simulink model "Main_Model_CB_EN_UEEE23112"  (R2025b)
settings: Solver=ode23t  StartTime=0.0  StopTime=25  MaxStep=1e-5  RelTol=1e-3  AbsTol=1e-4
values from neighbouring files (symbols this model uses):
  Tsc = 5e-5    (= 5e-05)    [Model_Parameters_CB_EN_U4EEE23112.m]
undefined symbols (not defined in the file or in its folder): dspblkCoreblockFVToolHelper, gcbh
libraries: nesl_utility x31, fl_lib x20, ee_lib x12, sdl_lib x4, batteryecm_lib x1, eePmsmFieldOrientedControl x1
(part 1 of 3)
settings Model: SimulationMode=accelerator  Creator=Hp  LastModifiedBy=Harish
settings SolverCC: AutoScaleAbsTol=off
settings ConfigComp: CovScope=ReferencedModels  CovMetricSettings=dzwe  CovHTMLOptions=-sRT=1 -sVT=0 -aTS=1 -agT=1 -bRG=1 -bTC=1 -hTR=0 -nFC=0 -nFD=0 -scm=1 -bcm=1 -xEv=0 -xEM=0 -req=1  CovEnableCumulative=off  CovCumulativeReport=on

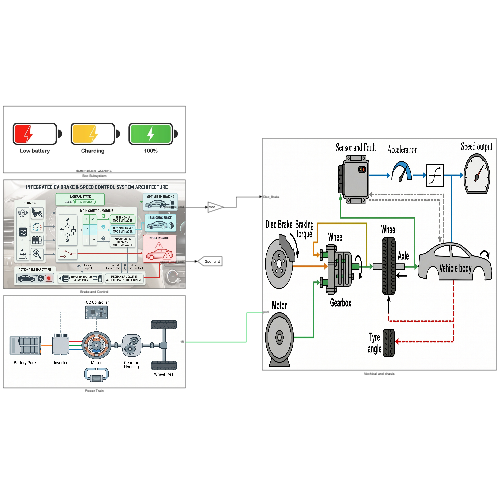
[thumbnail: Simulink's stored preview of the top-level diagram]
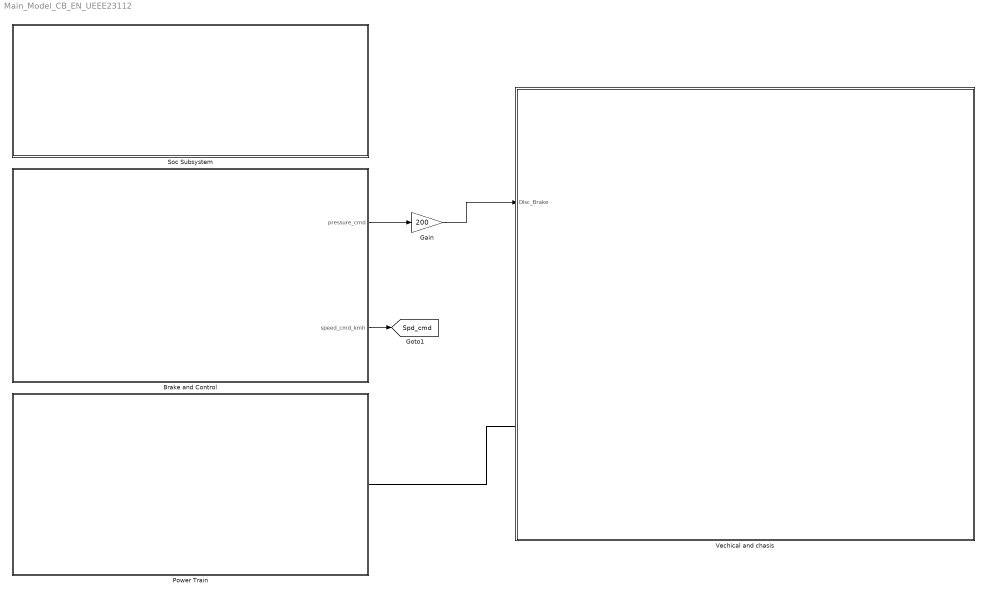
== system Main_Model_CB_EN_UEEE23112 ==
  Brake and Control : Subsystem
      mask Display: image('Brake_sub.png');
  Gain : Gain  Gain=200
  Power Train : Subsystem
      mask Display: image('Power_Train.png');
  Soc Subsystem : Subsystem
      mask Display: image('Soc.jpg');
  Vechical and chasis : Subsystem
      mask Display: image('Chasis.png');
  tag scope: Spd_cmd=global
  wires:
  Brake and Control/1(pressure_cmd) -> Gain/1
  Brake and Control/2(speed_cmd_kmh) -> [Spd_cmd]
  Gain/1 -> Vechical and chasis/1(Disc_Brake)
  connections:
  Power Train/RConn1 -- Vechical and chasis/LConn1

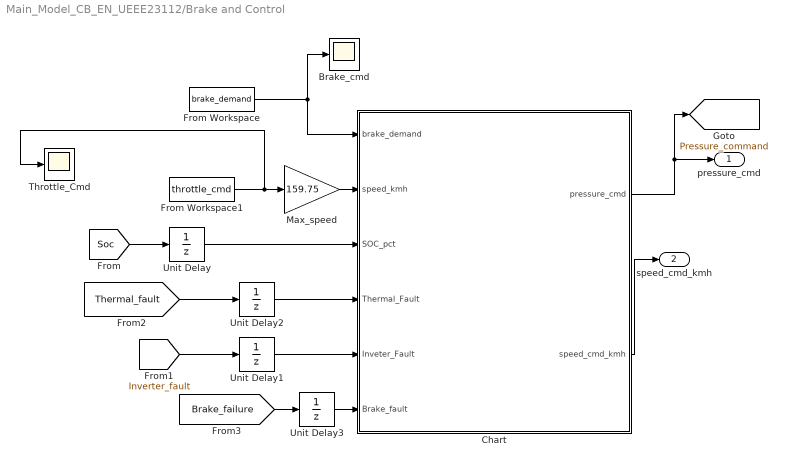
== system Main_Model_CB_EN_UEEE23112/Brake and Control ==
  Brake_cmd : Scope
      settings: ActiveDisplayYMinimum=-0.10624999999999997  ActiveDisplayYMaximum=0.95624999999999993  DataLoggingVariableName=ScopeData7
  Chart : Stateflow chart  TreatAsAtomicUnit=on
  From Workspace : FromWorkspace  VariableName=brake_demand  SampleTime=1e-4
  From Workspace1 : FromWorkspace  VariableName=throttle_cmd  SampleTime=1e-4
  Max_speed : Gain  Gain=159.75
  Throttle_Cmd : Scope
      settings: ActiveDisplayYMinimum=-0.049737499999999983  ActiveDisplayYMaximum=0.44763749999999997  DataLoggingVariableName=ScopeData8
  Unit Delay{,1..3} (4 alike) : UnitDelay  SampleTime=-1  HasFrameUpgradeWarning=on
  pressure_cmd : Outport
  speed_cmd_kmh : Outport  Port=2
  tag scope: Pressure_command=global
  wires:
  Chart/1(pressure_cmd) -> [Pressure_command], pressure_cmd/1
  Chart/2(speed_cmd_kmh) -> speed_cmd_kmh/1
  From Workspace1/1 -> Throttle_Cmd/1, Max_speed/1
  [Soc] -> Unit Delay/1
  From Workspace/1 -> Brake_cmd/1, Chart/1(brake_demand)
  Unit Delay/1 -> Chart/3(SOC_pct)
  Max_speed/1 -> Chart/2(speed_kmh)
  [Inverter_fault] -> Unit Delay1/1
  Unit Delay1/1 -> Chart/5(Inveter_Fault)
  [Thermal_fault] -> Unit Delay2/1
  Unit Delay2/1 -> Chart/4(Thermal_Fault)
  [Brake_failure] -> Unit Delay3/1
  Unit Delay3/1 -> Chart/6(Brake_fault)

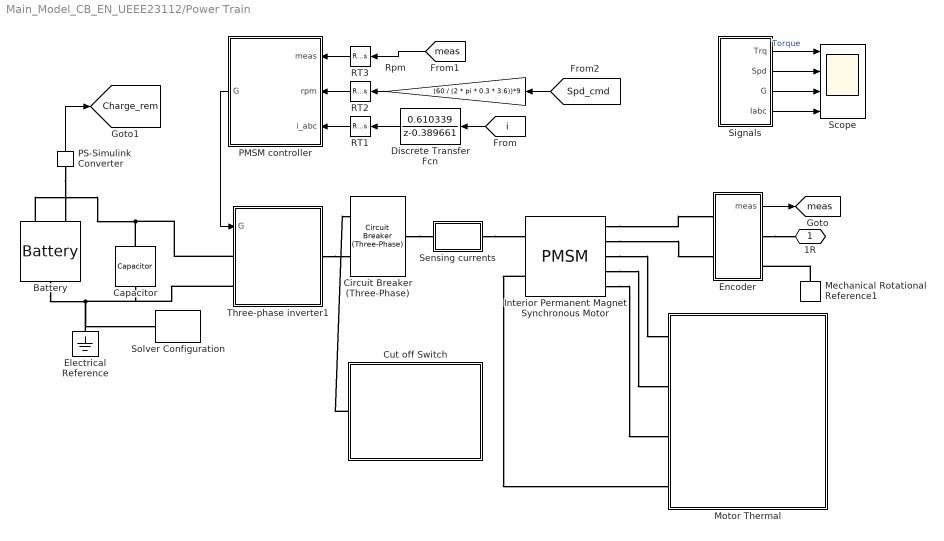
== system Main_Model_CB_EN_UEEE23112/Power Train ==
  Battery : batteryecm_lib/Battery  Vnom=800 V  prm_dir=simscape.enum.battery.prm_dir.enabled  R1_dis=0.05 Ohm  R1_ch=0.05 Ohm  R1=0.05 Ohm  prm_AH=simscape.enum.battery.prm_AH.finite  AH=75 hr*A  V1=720 V  AH1=8 hr*A  prm_R2=simscape.enum.battery.prm_R2.disabled  R2=inf Ohm  Tmeas=298.15 K  charge_measurement_port=simscape.enum.battery.enable.yes  prm_dyn=simscape.enum.battery.prm_dyn.off  Rp1=0.005 Ohm  tau1=30 s  Rp2=0.005 Ohm  tau2=30 s  Rp3=0.005 Ohm  tau3=30 s  Rp4=0.005 Ohm  tau4=30 s  Rp5=0.005 Ohm  tau5=30 s  prm_fade=simscape.enum.battery.prm_fade.enabled  N_fade=100  AH_fade=45 hr*A  R1_fade=2.02 Ohm  R1_ch_fade=2.02 Ohm  V1_fade=10.35 V  prm_age=simscape.enum.battery.prm_age.disabled  prm_age_OCV=1  OCV_age=0.9  SOC_age=60  Tmeas_age=298.15 K  delta_time_age_vec=[0] d  temperature_age_vec=[273] K  OCV_scaling_age=2.2134e6  OCV_offset_age=1.632e6  temp_exp_age=0.515833569 V  t_exp_age=0.75  Vnom_T2=12 V  R1_T2=2.2 Ohm  R1_T2_dis=2.2 Ohm  R1_T2_ch=2.2 Ohm  V1_T2=11.4 V  R2_T2=2200 Ohm  Rp1_T2=0.005 Ohm  tau1_T2=30 s  Rp2_T2=0.005 Ohm  tau2_T2=30 s  Rp3_T2=0.005 Ohm  tau3_T2=30 s  Rp4_T2=0.005 Ohm  tau4_T2=30 s  Rp5_T2=0.005 Ohm  tau5_T2=30 s  Tmeas2=273.15 K  thermal_port=simscape.enum.thermaleffects.omit  thermal_mass=30000 J/K  i_specify=off  i_priority=None  i=0 A  i_nominal_specify=off  i_nominal_value=1  i_nominal_unit=A  v_specify=off  v_priority=None  v=0 V  v_nominal_specify=off  v_nominal_value=1  v_nominal_unit=V  charge_specify=on  charge_priority=High  charge=65 hr*A  charge_nominal_specify=off  charge_nominal_value=1  charge_nominal_unit=A*hr  num_cycles_specify=off  num_cycles_priority=High  num_cycles=0  num_cycles_nominal_specify=off  num_cycles_nominal_value=1  num_cycles_nominal_unit=1  temperature_specify=off  temperature_priority=High  temperature=298.15 K  temperature_nominal_specify=off  temperature_nominal_value=1  temperature_nominal_unit=K
      settings: InternalSimscapePortConfiguration="{\"Bottom\":[],\"Left\":[{\"id\":\"p\",\"label\":\"+\",\"type\":\"foundation.electrical.electrical\"},{\"id\":\"q\",\"label\":\"q\",\"type\":\"output\"}],\"Right\":[{\"id\":\"n\",\"label\":\"-\",\"type\":\"foundation.electrical.electrical\"}],\"Top\":[]}"
  Capacitor : fl_lib/Electrical/Electrical Elements/Capacitor  c=1e-3 F  r=1e-6 Ohm  g=0 1/Ohm  i_specify=off  i_priority=None  i=0 A  i_nominal_specify=off  i_nominal_value=1  i_nominal_unit=A  v_specify=off  v_priority=None  v=0 V  v_nominal_specify=off  v_nominal_value=1  v_nominal_unit=V  vc_specify=off  vc_priority=High  vc=0 V  vc_nominal_specify=off  vc_nominal_value=1  vc_nominal_unit=V
  Circuit Breaker (Three-Phase) : ee_lib/Switches & Breakers/Circuit Breaker (Three-Phase)  R_closed=0.001 Ohm  G_open=1e-6 1/Ohm  threshold=0.5 V  breaker_behavior=ee.enum.switches.breakerBehavior.zeroCrossingDisable
      settings: InternalSimscapePortConfiguration="{\"Bottom\":[],\"Left\":[{\"id\":\"vT\",\"label\":\"vT\",\"type\":\"input\"},{\"id\":\"N1\",\"label\":\"~1\",\"type\":\"foundation.electrical.three_phase\"}],\"Right\":[{\"id\":\"N2\",\"label\":\"~2\",\"type\":\"foundation.electrical.three_phase\"}],\"Top\":[]}"
  Cut off Switch : Subsystem
      mask Display: image('Kill_switch_electrical.jpg');
  Discrete Transfer Fcn : DiscreteTransferFcn  LoadFcn=dspblkCoreblockFVToolHelper(gcbh,'load');  Numerator=[ 0.610339]  Denominator=[1, -0.389661]
      settings: CopyFcn=dspblkCoreblockFVToolHelper(gcbh,'copy');  DeleteFcn=dspblkCoreblockFVToolHelper(gcbh,'close');  ModelCloseFcn=dspblkCoreblockFVToolHelper(gcbh,'close');  PreSaveFcn=dspblkCoreblockFVToolHelper(gcbh,'presave');  PostSaveFcn=dspblkCoreblockFVToolHelper(gcbh,'postsave');  CloseFcn=dspblkCoreblockFVToolHelper(gcbh,'close');
  Electrical Reference : fl_lib/Electrical/Electrical Elements/Electrical Reference
  Encoder : Subsystem
  Interior Permanent Magnet Synchronous Motor : ee_lib/Electromechanical/Permanent Magnet/PMSM  port_option=ee.enum.threePhasePort.composite  winding_type=ee.enum.statorconnection.wye  machine_param=ee.enum.pmsm.parameterization.constant  nPolePairs=4  pmflux_param=ee.enum.pmflux.fluxlinkage  pm_flux_linkage=0.05 Wb  torque_constant=0.18 N*m/A  back_emf_constant=0.18 V/(rad/s)  stator_param=ee.enum.statorparam.LdLqL0  Ld=0.00013 H  Lq=0.00038 H  idVec=[-200, 0, 200] A  iqVec=[-200, 0, 200] A  LdMatrix=0.0002 * ones(3, 3) H  LqMatrix=0.0002 * ones(3, 3) H  PmMatrix=0.1 * ones(3, 3) Wb  ktMatrix=0.18 * ones(3, 3) N*m/A  keMatrix=0.18 * ones(3, 3) V/(rad/s)  L0=L0 H  Ls=0.0002 H  Lm=0.00002 H  Ms=0.00002 H  Rs=0.01 Ohm  zero_sequence=ee.enum.park.zerosequence.exclude  axes_param=ee.enum.rotorangle.qaxis  loss_param=ee.enum.ironloss.none  losses_oc=[0, 0, 0] W  losses_sc=[0, 0, 0] W  f_losses=60 Hz  Isc_losses=95 A  J=0 kg*m^2  lam=0 N*m/(rad/s)  i_d_specify=off  i_d_priority=None  i_d=0 A  i_d_nominal_specify=off  i_d_nominal_value=1  i_d_nominal_unit=A  i_q_specify=off  i_q_priority=None  i_q=0 A  i_q_nominal_specify=off  i_q_nominal_value=1  i_q_nominal_unit=A  torque_specify=off  torque_priority=None  torque=0 N*m  torque_nominal_specify=off  torque_nominal_value=1  torque_nominal_unit=N*m  angular_velocity_specify=on  angular_velocity_priority=None  angular_velocity=0 rpm  angular_velocity_nominal_specify=off  angular_velocity_nominal_value=1  angular_velocity_nominal_unit=rpm  angular_position_specify=on  angular_position_priority=High  angular_position=0 rad  angular_position_nominal_specify=off  angular_position_nominal_value=1  angular_position_nominal_unit=deg  alpha=3.93e-3 1/K  alpha_flux=-0.001 1/K  Tmeas=298.15 K  stator_thermal_mass=20000 J/K  rotor_thermal_mass=7500 J/K  Rm_percent_rotor=90  Rd_percent_rotor=30  temperatureA_specify=off  temperatureA_priority=High  temperatureA=25 degC  temperatureA_nominal_specify=off  temperatureA_nominal_value=1  temperatureA_nominal_unit=degC  temperatureB_specify=off  temperatureB_priority=High  temperatureB=25 degC  temperatureB_nominal_specify=off  temperatureB_nominal_value=1  temperatureB_nominal_unit=degC  temperatureC_specify=off  temperatureC_priority=High  temperatureC=25 degC  temperatureC_nominal_specify=off  temperatureC_nominal_value=1  temperatureC_nominal_unit=degC  temperatureR_specify=off  temperatureR_priority=High  temperatureR=25 degC  temperatureR_nominal_specify=off  temperatureR_nominal_value=1  temperatureR_nominal_unit=degC
      settings: InternalSimscapePortConfiguration="{\"Bottom\":[],\"Left\":[{\"id\":\"N\",\"label\":\"~\",\"type\":\"foundation.electrical.three_phase\"},{\"id\":\"HR\",\"label\":\"HR\",\"type\":\"foundation.thermal.thermal\"}],\"Right\":[{\"id\":\"R\",\"label\":\"R\",\"type\":\"foundation.mechanical.rotational.rotational\"},{\"id\":\"C\",\"label\":\"C\",\"type\":\"foundation.mechanical.rotational.rotational\"},{\"id\":\"HA\",\"label\":\"HA\",\"type\":\"foundation.thermal.thermal\"},{\"id\":\"HB\",\"label\":\"HB\",\"type\":\"foundation.thermal.thermal\"},{\"id\":\"HC\",\"label\":\"HC\",\"type\":\"foundation.thermal.thermal\"}],\"Top\":[]}"
  Mechanical Rotational Reference1 : fl_lib/Mechanical/Rotational Elements/Mechanical Rotational Reference
  Motor Thermal : Subsystem
      mask Display: image('Temp.png');
  PMSM controller : Subsystem
      mask Display: image('Foc_controller.jpg');
  PS-Simulink Converter : nesl_utility/PS-Simulink Converter  PhysicalDomain=network_engine_domain  SubClassName=ps_output  LeftPortType=input  RightPortType=output  PseudoPeriodic=off  Frequencies=[]  VectorFormat=inherit  Unit=inherit  AffineConversion=off
  RT1 : RateTransition  OutPortSampleTime=Tsc
  RT2 : RateTransition  OutPortSampleTime=Tsc
  RT3 : RateTransition  OutPortSampleTime=Tsc
  Rpm : Gain  Gain=(60 / (2 * pi * 0.3 * 3.6))*9
  Scope : Scope  NumInputPorts=4
      settings: SampleTime=5e-6  Title=Demanded and achieved torques  ActiveDisplayYMinimum=-415.91098780248285  ActiveDisplayYMaximum=394.62396867045919  DataLoggingVariableName=ScopeData3
  Sensing currents : Subsystem
      mask Display: disp('i')
  "Signals " : Subsystem
  Solver Configuration : nesl_utility/Solver Configuration  PhysicalDomain=network_engine_domain  SubClassName=solver  LeftPortType=input  RightPortType=generic  Tones=[]  Harmonics=[]  SimulateNoise=off  Profile=off  UseLocalSampling=off  EnableSwitchedLinearOptims=on  FrequencyDomain=off  UseCCode=off  RelTol=0.001  AbsTol=0.001  MinStep=1e-09  ToWorkspace=off  RevertToSquareIcSolve=off  NumHomotopyIterations=100  PhasorMode=off  PhasorModeNumHarmonics=1  ConsistencySolver=NEWTON_XTOL_AFTER_FTOL  IndexReductionMethod=DerivativeReplacement  DoDC=off  ResidualTolerance=1e-09  ConsistencyTolSource=GLOBAL  ConsistencyAbsTol=0.001  ConsistencyRelTol=0.001  ConsistencyTolFactor=0.001  UseLocalSolver=off  LocalSolverChoice=NE_BACKWARD_EULER_ADVANCER  ResolveIndetEquations=on  FunctionEvalNumThread=1  LocalSolverSampleTime=0.001  DoFixedCost=off  MaxNonlinIter=3  MaxModeIter=2  ComputeImpulses=off  ImpulseIterations=2  LinearAlgebra=auto  LinearAlgebraNumThread=0  EquationFormulation=NE_TIME_EF  DelaysMemoryBudget=1024  AutomaticFiltering=on  FilteringTimeConstant=0.001  PartitionStorageMethod=AS_NEEDED  PartitionMemoryBudget=1024  PartitionMethod=ROBUST  MultibodyUseLocalSolver=off  MultibodyLocalSolverChoice=ODE1  MultibodyLocalSolverSampleTime=0.001
  Three-phase inverter1 : Subsystem
      mask Display: image('Inverter.jpg');
  1R : PMIOPort  Side=Right
  tag scope: Charge_rem=global, meas=global
  wires:
  Encoder/1(meas) -> [meas]
  "Signals "/1(Trq) -> Scope/1  "Torque"
  RT2/1 -> PMSM controller/2(rpm)
  RT1/1 -> PMSM controller/3(i_abc)
  RT3/1 -> PMSM controller/1(meas)
  "Signals "/4(Iabc) -> Scope/4
  [meas] -> RT3/1
  "Signals "/2(Spd) -> Scope/2
  PMSM controller/1(G) -> Three-phase inverter1/1(G)
  "Signals "/3(G) -> Scope/3
  [i] -> Discrete Transfer Fcn/1
  Discrete Transfer Fcn/1 -> RT1/1
  Rpm/1 -> RT2/1
  PS-Simulink Converter/1 -> [Charge_rem]
  [Spd_cmd] -> Rpm/1
  connections:
  Battery/LConn1 -- Three-phase inverter1/LConn1 -- Capacitor/LConn1
  Interior Permanent Magnet Synchronous Motor/RConn2 -- Encoder/LConn2
  Battery/RConn1 -- Solver Configuration/RConn1 -- Electrical Reference/LConn1 -- Three-phase inverter1/LConn2 -- Capacitor/RConn1
  Mechanical Rotational Reference1/LConn1 -- Encoder/RConn2
  Encoder/RConn1 -- 1R/RConn1
  Interior Permanent Magnet Synchronous Motor/RConn1 -- Encoder/LConn1
  PS-Simulink Converter/LConn1 -- Battery/LConn2
  Interior Permanent Magnet Synchronous Motor/LConn2 -- Motor Thermal/LConn4
  Sensing currents/RConn1 -- Interior Permanent Magnet Synchronous Motor/LConn1
  Three-phase inverter1/RConn1 -- Circuit Breaker (Three-Phase)/LConn2
  Circuit Breaker (Three-Phase)/RConn1 -- Sensing currents/LConn1
  Interior Permanent Magnet Synchronous Motor/RConn3 -- Motor Thermal/LConn1
  Interior Permanent Magnet Synchronous Motor/RConn4 -- Motor Thermal/LConn2
  Interior Permanent Magnet Synchronous Motor/RConn5 -- Motor Thermal/LConn3
  Cut off Switch/RConn1 -- Circuit Breaker (Three-Phase)/LConn1

== system Main_Model_CB_EN_UEEE23112/Soc Subsystem ==
  Constant1 : Constant  Value=25.2e6
  Divide : Product  Inputs=*/
  Percent : Gain  Gain=100
  Soc : Scope
      settings: ActiveDisplayYMinimum=0.92713614673266553  ActiveDisplayYMaximum=0.92747057637032393  DataLoggingVariableName=ScopeData2
  tag scope: Soc=global
  wires:
  [Charge_rem] -> Divide/1
  Percent/1 -> [Soc], Soc/1
  Divide/1 -> Percent/1
  Constant1/1 -> Divide/2

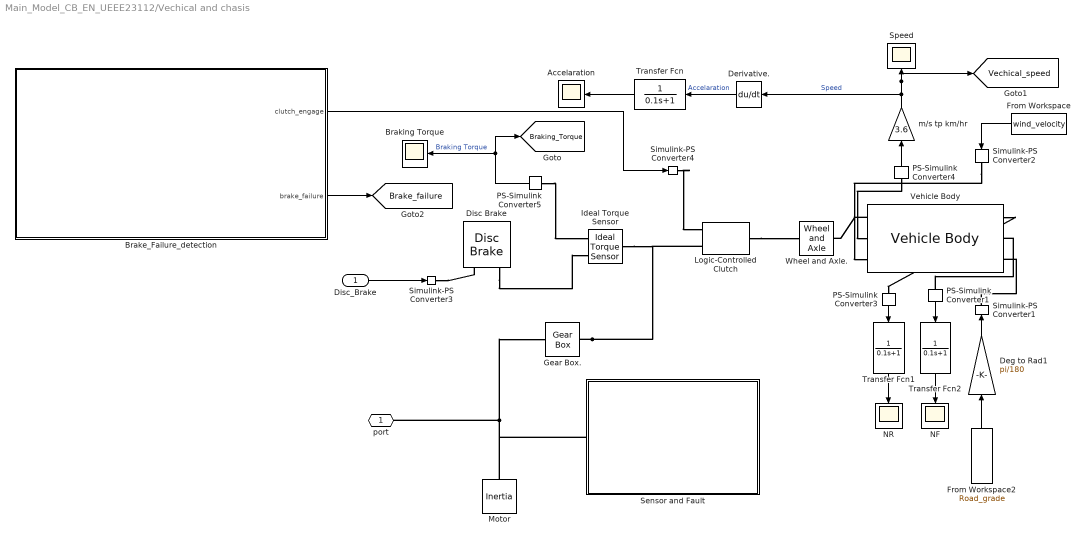
== system Main_Model_CB_EN_UEEE23112/Vechical and chasis ==
  Disc_Brake : Inport
  Accelaration : Scope
      settings: ActiveDisplayYMinimum=-27.27425273691172  ActiveDisplayYMaximum=13.251308134917883
  Brake_Failure_detection : Subsystem
      mask Display: image('Brake_failure.jpeg');
  Braking Torque : Scope
      settings: ActiveDisplayYMinimum=-1  ActiveDisplayYMaximum=1  DataLoggingVariableName=ScopeData25
  Deg to Rad1 : Gain  Gain=pi/180
  Derivative. : Derivative
  Disc Brake : sdl_lib/Brakes & Detents/Rotational/Disc Brake  r_mean=150 mm  bore=40 mm  n_pads=2  thermal_port=simscape.enum.thermaleffects.omit  mu_static=0.9  mu_coulomb=0.7  temperature_TLU=[280, 300, 320] K  mu_static_TLU=[.9, .8, .7]  mu_coulomb_TLU=[.8, .7, .6]  brkwy_vel=0.1 rad/s  visc_coef=0 N*m*s/rad  thermal_mass=50 kJ/K  temperature_specify=off  temperature_priority=High  temperature=300 K  temperature_nominal_specify=off  temperature_nominal_value=1  temperature_nominal_unit=K
  From Workspace : FromWorkspace  VariableName=wind_velocity
  From Workspace2 : FromWorkspace  VariableName=Road_grade  OutDataTypeStr=double  OutputAfterFinalValue=Setting to zero
  Gear Box. : fl_lib/Mechanical/Mechanisms/Gear Box  ratio=9  t_in_specify=off  t_in_priority=None  t_in=0 N*m  t_in_nominal_specify=off  t_in_nominal_value=1  t_in_nominal_unit=N*m  t_out_specify=off  t_out_priority=None  t_out=0 N*m  t_out_nominal_specify=off  t_out_nominal_value=1  t_out_nominal_unit=N*m
  Ideal Torque Sensor : fl_lib/Mechanical/Mechanical Sensors/Ideal Torque Sensor
  Logic-Controlled Clutch : sdl_lib/Clutches/Logic-Controlled Clutch  transition_model=sdl.enum.transitionModel.instant  transition_time_constant=0.1 s  t_friction=2500 N*m  t_locked=3200 N*m  w_tol=0.01 rad/s  initial_state_locked=sdl.enum.initial_lock.locked
      settings: InternalSimscapePortConfiguration="{\"Bottom\":[],\"Left\":[{\"id\":\"E\",\"label\":\"E\",\"type\":\"input\"},{\"id\":\"B\",\"label\":\"B\",\"type\":\"foundation.mechanical.rotational.rotational\"}],\"Right\":[{\"id\":\"F\",\"label\":\"F\",\"type\":\"foundation.mechanical.rotational.rotational\"}],\"Top\":[]}"
  Motor : fl_lib/Mechanical/Rotational Elements/Inertia  inertia=0.100 kg*m^2  num_ports=foundation.enum.numPorts2.one  w_specify=off  w_priority=High  w=0 rad/s  w_nominal_specify=off  w_nominal_value=1  w_nominal_unit=rad/s  t_specify=off  t_priority=None  t=0 N*m  t_nominal_specify=off  t_nominal_value=1  t_nominal_unit=N*m
  NF : Scope
      settings: ActiveDisplayYMinimum=-439.89583333262539  ActiveDisplayYMaximum=3959.0624999936294  DataLoggingVariableName=ScopeData4
  NR : Scope
      settings: ActiveDisplayYMinimum=-1  ActiveDisplayYMaximum=1  DataLoggingVariableName=ScopeData5
  PS-Simulink Converter{1,3..5} (4 alike) : nesl_utility/PS-Simulink Converter  PhysicalDomain=network_engine_domain  SubClassName=ps_output  LeftPortType=input  RightPortType=output  PseudoPeriodic=off  Frequencies=[]  VectorFormat=inherit  Unit=inherit  AffineConversion=off
  Sensor and Fault : Subsystem
      mask Display: image('speed_sensor.jpg');
  Simulink-PS Converter{1..4} (4 alike) : nesl_utility/Simulink-PS Converter  PhysicalDomain=network_engine_domain  SubClassName=ps_input  LeftPortType=input  RightPortType=output  PseudoPeriodic=off  Frequencies=[]  NoiseDistribution=none  NoiseParameters=[]  Unit=1  AffineConversion=off  FilteringAndDerivatives=provide  SimscapeFilterOrder=1  InputFilterTimeConstant=0.001  UdotUserProvided=0
  Speed : Scope
      settings: ActiveDisplayYMinimum=-8.0401114234250759  ActiveDisplayYMaximum=72.360918458878444  DataLoggingVariableName=ScopeData6
  Transfer Fcn : TransferFcn  Denominator=[0.1 1]
  Transfer Fcn1 : TransferFcn  Denominator=[0.1 1]
  Transfer Fcn2 : TransferFcn  Denominator=[0.1 1]
  Vehicle Body : sdl_lib/Tires & Vehicles/Vehicle Body  mass=1200 kg  n_w=2  x_f=a_cg m  x_r=b_cg m  y_c=h_cg m  mass_var=false  g=9.81 m/s^2  liftoff_warning=false  area=2 m^2  Cd_var=false  Cd=0.3  rho=1.18 kg/m^3  model_pitch=false  inertia=4000 kg*m^2  suspension_model=sdl.enum.linearTLU.linear  k_f=1e4 N/m  b_f=1e4 N*s/m  k_r=1e4 N/m  b_r=1e4 N*s/m  k_f_TLU=[-2000, -1000, 0, 1000, 2000] N  x_f_TLU=[-.4, -.2, 0, .2, .4] m  b_f_TLU=[-200, -100, 0, 100, 200] N  v_f_TLU=[-4, -2, 0, 2, 4] m/s  k_r_TLU=[-2000, -1000, 0, 1000, 2000] N  x_r_TLU=[-.4, -.2, 0, .2, .4] m  b_r_TLU=[-200, -100, 0, 100, 200] N  v_r_TLU=[-4, -2, 0, 2, 4] m/s  interp_method=simscape.enum.interpolation.linear  extrap_method=simscape.enum.extrapolation.linear  model_hardstop=false  upper_bound_f=.25 m  lower_bound_f=-.25 m  stop_k_f=1e6 N/m  stop_b_f=150 N*s/m  upper_bound_r=.25 m  lower_bound_r=-.25 m  stop_k_r=1e6 N/m  stop_b_r=150 N*s/m  initial_pitch=0 rad  initial_pitch_rate=0 rad/s  v_specify=on  v_priority=High  v=0 m/s  v_nominal_specify=off  v_nominal_value=1  v_nominal_unit=m/s
      settings: InternalSimscapePortConfiguration="{\"Bottom\":[{\"id\":\"NR\",\"label\":\"NR\",\"type\":\"output\"},{\"id\":\"NF\",\"label\":\"NF\",\"type\":\"output\"},{\"id\":\"beta\",\"label\":\"beta\",\"type\":\"input\"}],\"Left\":[{\"id\":\"H\",\"label\":\"H\",\"type\":\"foundation.mechanical.translational.translational\"}],\"Right\":[],\"Top\":[{\"id\":\"V\",\"label\":\"V\",\"type\":\"output\"},{\"id\":\"wind\",\"label\":\"W\",\"type\":\"input\"}]}"
  Wheel and Axle. : fl_lib/Mechanical/Mechanisms/Wheel and Axle  R=0.30 m  or=1  t_specify=off  t_priority=None  t=0 N*m  t_nominal_specify=off  t_nominal_value=1  t_nominal_unit=N*m  f_specify=off  f_priority=None  f=0 N  f_nominal_specify=off  f_nominal_value=1  f_nominal_unit=N
  m/s tp km/hr : Gain  Gain=3.6
  port : PMIOPort  Side=Left
  tag scope: Brake_failure=global, Braking_Torque=global, Vechical_speed=global
  wires:
  PS-Simulink Converter3/1 -> Transfer Fcn1/1
  Transfer Fcn2/1 -> NF/1
  m/s tp km/hr/1 -> [Vechical_speed], Speed/1, Derivative./1  "Speed"
  Derivative./1 -> Transfer Fcn/1  "Accelaration"
  PS-Simulink Converter4/1 -> m/s tp km/hr/1
  PS-Simulink Converter1/1 -> Transfer Fcn2/1
  Disc_Brake/1 -> Simulink-PS Converter3/1
  From Workspace2/1 -> Deg to Rad1/1
  Transfer Fcn1/1 -> NR/1
  Transfer Fcn/1 -> Accelaration/1
  Deg to Rad1/1 -> Simulink-PS Converter1/1
  PS-Simulink Converter5/1 -> [Braking_Torque], Braking Torque/1  "Braking Torque"
  Brake_Failure_detection/1(clutch_engage) -> Simulink-PS Converter4/1
  Brake_Failure_detection/2(brake_failure) -> [Brake_failure]
  From Workspace/1 -> Simulink-PS Converter2/1
  connections:
  Vehicle Body/RConn1 -- PS-Simulink Converter3/LConn1
  PS-Simulink Converter1/LConn1 -- Vehicle Body/RConn2
  PS-Simulink Converter4/LConn1 -- Vehicle Body/LConn2
  Simulink-PS Converter1/RConn1 -- Vehicle Body/RConn3
  Simulink-PS Converter3/RConn1 -- Disc Brake/LConn1
  Vehicle Body/LConn1 -- Wheel and Axle./RConn1
  Simulink-PS Converter2/RConn1 -- Vehicle Body/LConn3
  PS-Simulink Converter5/LConn1 -- Ideal Torque Sensor/RConn2
  Disc Brake/LConn2 -- Ideal Torque Sensor/RConn1
  Gear Box./RConn1 -- Logic-Controlled Clutch/LConn2 -- Ideal Torque Sensor/LConn1
  Logic-Controlled Clutch/RConn1 -- Wheel and Axle./LConn1
  Simulink-PS Converter4/RConn1 -- Logic-Controlled Clutch/LConn1
  Motor/LConn1 -- Sensor and Fault/LConn1 -- Gear Box./LConn1 -- port/RConn1

== system Main_Model_CB_EN_UEEE23112/Power Train/Cut off Switch ==
  Data Type Conversion : DataTypeConversion  OutDataTypeStr=double  SaturateOnIntegerOverflow=off  RndMeth=Floor
  Logical Operator : Logic  Operator=OR  AllPortsSameDT=off  OutDataTypeStr=boolean
  Simulink-PS Converter : nesl_utility/Simulink-PS Converter  PhysicalDomain=network_engine_domain  SubClassName=ps_input  LeftPortType=input  RightPortType=output  PseudoPeriodic=off  Frequencies=[]  NoiseDistribution=none  NoiseParameters=[]  Unit=1  AffineConversion=off  FilteringAndDerivatives=provide  SimscapeFilterOrder=1  InputFilterTimeConstant=0.001  UdotUserProvided=0
  Unit Delay : UnitDelay  SampleTime=-1  HasFrameUpgradeWarning=on
  Unit Delay1 : UnitDelay  SampleTime=-1  HasFrameUpgradeWarning=on
  output : PMIOPort  Side=Right
  wires:
  Logical Operator/1 -> Data Type Conversion/1
  [Inverter_fault] -> Unit Delay1/1
  [Thermal_fault] -> Unit Delay/1
  Data Type Conversion/1 -> Simulink-PS Converter/1
  Unit Delay/1 -> Logical Operator/2
  Unit Delay1/1 -> Logical Operator/1
  connections:
  Simulink-PS Converter/RConn1 -- output/RConn1

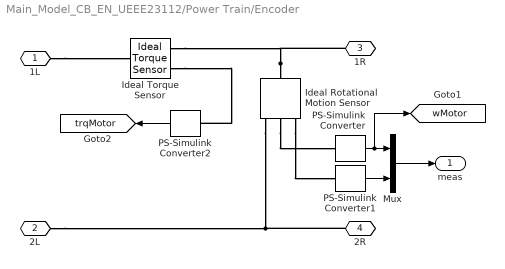
== system Main_Model_CB_EN_UEEE23112/Power Train/Encoder ==
  Ideal Rotational Motion Sensor : fl_lib/Mechanical/Mechanical Sensors/Ideal Rotational Motion Sensor  reference=foundation.enum.MeasurementReference.difference  acceleration_port=false  velocity_port=true  position_port=true  wrap_angle=simscape.enum.onoff.off  offset=0 deg
  Ideal Torque Sensor : fl_lib/Mechanical/Mechanical Sensors/Ideal Torque Sensor
  Mux : Mux  Inputs=2
  PS-Simulink Converter : nesl_utility/PS-Simulink Converter  PhysicalDomain=network_engine_domain  SubClassName=ps_output  LeftPortType=input  RightPortType=output  PseudoPeriodic=off  Frequencies=[]  VectorFormat=1-D array  Unit=rad/s  AffineConversion=off
  PS-Simulink Converter1 : nesl_utility/PS-Simulink Converter  PhysicalDomain=network_engine_domain  SubClassName=ps_output  LeftPortType=input  RightPortType=output  PseudoPeriodic=off  Frequencies=[]  VectorFormat=1-D array  Unit=rad  AffineConversion=off
  PS-Simulink Converter2 : nesl_utility/PS-Simulink Converter  PhysicalDomain=network_engine_domain  SubClassName=ps_output  LeftPortType=input  RightPortType=output  PseudoPeriodic=off  Frequencies=[]  VectorFormat=1-D array  Unit=N*m  AffineConversion=off
  1L : PMIOPort  Side=Left
  2L : PMIOPort  Port=2  Side=Left
  1R : PMIOPort  Port=3  Side=Right
  2R : PMIOPort  Port=4  Side=Right
  meas : Outport  VectorParamsAs1DForOutWhenUnconnected=off
  tag scope: trqMotor=global, wMotor=global
  wires:
  PS-Simulink Converter2/1 -> [trqMotor]
  Mux/1 -> meas/1
  PS-Simulink Converter1/1 -> Mux/2
  PS-Simulink Converter/1 -> [wMotor], Mux/1
  connections:
  Ideal Torque Sensor/RConn2 -- PS-Simulink Converter2/LConn1
  1L/RConn1 -- Ideal Torque Sensor/LConn1
  2R/RConn1 -- 2L/RConn1 -- Ideal Rotational Motion Sensor/RConn1
  Ideal Rotational Motion Sensor/LConn1 -- 1R/RConn1 -- Ideal Torque Sensor/RConn1
  Ideal Rotational Motion Sensor/RConn2 -- PS-Simulink Converter/LConn1
  Ideal Rotational Motion Sensor/RConn3 -- PS-Simulink Converter1/LConn1

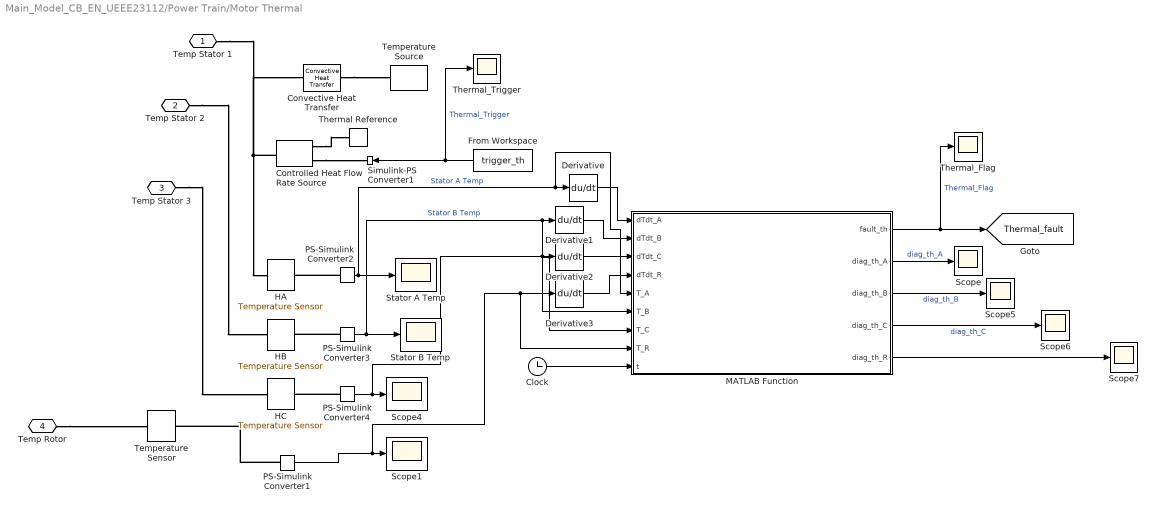
== system Main_Model_CB_EN_UEEE23112/Power Train/Motor Thermal ==
  Clock : Clock
  Controlled Heat Flow Rate Source : fl_lib/Thermal/Thermal Sources/Controlled Heat Flow Rate Source
  Convective Heat Transfer : fl_lib/Thermal/Thermal Elements/Convective Heat Transfer  thermal_type=foundation.enum.constant_variable.constant  area=1 m^2  heat_tr_coeff=5000 W/(K*m^2)  min_heat_tr_coeff=1e-3 W/(K*m^2)  T_specify=off  T_priority=None  T=0 K  T_nominal_specify=off  T_nominal_value=1  T_nominal_unit=K  Q_specify=off  Q_priority=None  Q=0 W  Q_nominal_specify=off  Q_nominal_value=1  Q_nominal_unit=W
  Derivative{,1..3} (4 alike) : Derivative
  From Workspace : FromWorkspace  VariableName=trigger_th
  HA : fl_lib/Thermal/Thermal Sensors/Temperature Sensor  temperature_measure=foundation.enum.MeasurementReference.absolute
      settings: InternalSimscapePortConfiguration="{\"Bottom\":[],\"Left\":[{\"id\":\"A\",\"label\":\"A\",\"type\":\"foundation.thermal.thermal\"}],\"Right\":[{\"id\":\"T\",\"label\":\"T\",\"type\":\"output\"}],\"Top\":[]}"
  HB : fl_lib/Thermal/Thermal Sensors/Temperature Sensor  temperature_measure=foundation.enum.MeasurementReference.absolute
      settings: InternalSimscapePortConfiguration="{\"Bottom\":[],\"Left\":[{\"id\":\"A\",\"label\":\"A\",\"type\":\"foundation.thermal.thermal\"}],\"Right\":[{\"id\":\"T\",\"label\":\"T\",\"type\":\"output\"}],\"Top\":[]}"
  HC : fl_lib/Thermal/Thermal Sensors/Temperature Sensor  temperature_measure=foundation.enum.MeasurementReference.absolute
      settings: InternalSimscapePortConfiguration="{\"Bottom\":[],\"Left\":[{\"id\":\"A\",\"label\":\"A\",\"type\":\"foundation.thermal.thermal\"}],\"Right\":[{\"id\":\"T\",\"label\":\"T\",\"type\":\"output\"}],\"Top\":[]}"
  MATLAB Function : MATLAB Function  TreatAsAtomicUnit=on
  PS-Simulink Converter{1..4} (4 alike) : nesl_utility/PS-Simulink Converter  PhysicalDomain=network_engine_domain  SubClassName=ps_output  LeftPortType=input  RightPortType=output  PseudoPeriodic=off  Frequencies=[]  VectorFormat=inherit  Unit=inherit  AffineConversion=off
  Scope{,1,4..7} (6 alike) : Scope
      Scope settings: ActiveDisplayYMinimum=-0.12499999999999997  ActiveDisplayYMaximum=1.125  DataLoggingVariableName=ScopeData19
      Scope1 settings: ActiveDisplayYMinimum=-1  ActiveDisplayYMaximum=1  DataLoggingVariableName=ScopeData9
      Scope4 settings: ActiveDisplayYMinimum=-1  ActiveDisplayYMaximum=1  DataLoggingVariableName=ScopeData12
      Scope5 settings: ActiveDisplayYMinimum=-1  ActiveDisplayYMaximum=1  DataLoggingVariableName=ScopeData20
      Scope6 settings: ActiveDisplayYMinimum=-1  ActiveDisplayYMaximum=1  DataLoggingVariableName=ScopeData21
      Scope7 settings: ActiveDisplayYMinimum=-1  ActiveDisplayYMaximum=1  DataLoggingVariableName=ScopeData22
  Simulink-PS Converter1 : nesl_utility/Simulink-PS Converter  PhysicalDomain=network_engine_domain  SubClassName=ps_input  LeftPortType=input  RightPortType=output  PseudoPeriodic=off  Frequencies=[]  NoiseDistribution=none  NoiseParameters=[]  Unit=1  AffineConversion=off  FilteringAndDerivatives=filter  SimscapeFilterOrder=1  InputFilterTimeConstant=1e-4  UdotUserProvided=0
  Stator A Temp : Scope
      settings: ActiveDisplayYMinimum=296.80419816376065  ActiveDisplayYMaximum=310.26221652615408  DataLoggingVariableName=ScopeData10
  Stator B Temp : Scope
      settings: ActiveDisplayYMinimum=298.09175430595883  ActiveDisplayYMaximum=298.67421124637036  DataLoggingVariableName=ScopeData11
  Temperature Sensor : fl_lib/Thermal/Thermal Sensors/Temperature Sensor  temperature_measure=foundation.enum.MeasurementReference.absolute
      settings: InternalSimscapePortConfiguration="{\"Bottom\":[],\"Left\":[{\"id\":\"A\",\"label\":\"A\",\"type\":\"foundation.thermal.thermal\"}],\"Right\":[{\"id\":\"T\",\"label\":\"T\",\"type\":\"output\"}],\"Top\":[]}"
  Temperature Source : fl_lib/Thermal/Thermal Sources/Temperature Source  temperature=298.15 K
  Thermal Reference : fl_lib/Thermal/Thermal Elements/Thermal Reference
  Thermal_Flag : Scope
      settings: ActiveDisplayYMinimum=-0.12499999999999997  ActiveDisplayYMaximum=1.125  DataLoggingVariableName=ScopeData24
  Thermal_Trigger : Scope
      settings: ActiveDisplayYMinimum=-62499.999999999985  ActiveDisplayYMaximum=562500  DataLoggingVariableName=ScopeData23
  Temp Stator 1 : PMIOPort  Side=Left
  Temp Stator 2 : PMIOPort  Port=2  Side=Left
  Temp Stator 3 : PMIOPort  Port=3  Side=Left
  "Temp Rotor " : PMIOPort  Port=4  Side=Left
  tag scope: Thermal_fault=global
  wires:
  PS-Simulink Converter4/1 -> MATLAB Function/7(T_C), Derivative2/1, Scope4/1
  PS-Simulink Converter3/1 -> Stator B Temp/1, MATLAB Function/6(T_B), Derivative1/1  "Stator B Temp"
  From Workspace/1 -> Thermal_Trigger/1, Simulink-PS Converter1/1  "Thermal_Trigger"
  PS-Simulink Converter2/1 -> Stator A Temp/1, MATLAB Function/5(T_A), Derivative/1  "Stator A Temp"
  PS-Simulink Converter1/1 -> Derivative3/1, MATLAB Function/8(T_R), Scope1/1
  Derivative/1 -> MATLAB Function/1(dTdt_A)
  Clock/1 -> MATLAB Function/9(t)
  MATLAB Function/1(fault_th) -> Thermal_Flag/1, [Thermal_fault]  "Thermal_Flag"
  MATLAB Function/2(diag_th_A) -> Scope/1  "diag_th_A"
  MATLAB Function/3(diag_th_B) -> Scope5/1  "diag_th_B"
  MATLAB Function/4(diag_th_C) -> Scope6/1  "diag_th_C"
  MATLAB Function/5(diag_th_R) -> Scope7/1
  Derivative1/1 -> MATLAB Function/2(dTdt_B)
  Derivative2/1 -> MATLAB Function/3(dTdt_C)
  Derivative3/1 -> MATLAB Function/4(dTdt_R)
  connections:
  PS-Simulink Converter4/LConn1 -- HC/RConn1
  Controlled Heat Flow Rate Source/LConn1 -- Temp Stator 1/RConn1 -- Convective Heat Transfer/LConn1 -- HA/LConn1
  PS-Simulink Converter2/LConn1 -- HA/RConn1
  PS-Simulink Converter3/LConn1 -- HB/RConn1
  Controlled Heat Flow Rate Source/RConn1 -- Simulink-PS Converter1/RConn1
  Controlled Heat Flow Rate Source/RConn2 -- Thermal Reference/LConn1
  Temp Stator 3/RConn1 -- HC/LConn1
  Temp Stator 2/RConn1 -- HB/LConn1
  PS-Simulink Converter1/LConn1 -- Temperature Sensor/RConn1
  "Temp Rotor "/RConn1 -- Temperature Sensor/LConn1
  Convective Heat Transfer/RConn1 -- Temperature Source/LConn1

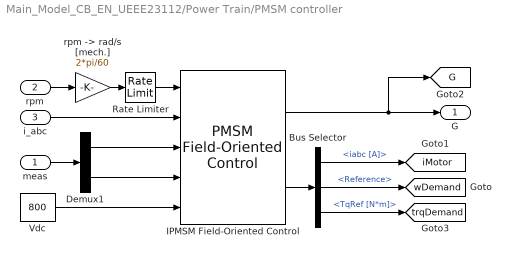
== system Main_Model_CB_EN_UEEE23112/Power Train/PMSM controller ==
  meas : Inport
  rpm : Inport  Port=2
  i_abc : Inport  Port=3
  Bus Selector : BusSelector  OutputSignals=iabc [A],Reference,TqRef [N*m]
  Demux1 : Demux  Outputs=2
  IPMSM Field-Oriented Control : eePmsmFieldOrientedControl/PMSM Field-Oriented Control  winding_type=Wye-wound  CtrlMode=Velocity control  Vnom=800  Pmax=106e3  Tmax=250  p=4  Vdc_on=10  Ts=5e-6  Tsc=5e-5  CtrlType=PI control  Kp_w=8  Ki_w=15  Kv_w=1  Kaw_w=10  RefType=Lookup-table based  rpmVec=[0:100:12000];  TqVec=[-250:2:250]  VdcVec=[700,750, 800];  PWMMode=SVM: space vector modulation  ModFactor=1  idMatrix=id_LUT  iqMatrix=iq_LUT  psim=0.05  Ld=0.00015  Lq=0.00045  Rs=0.01  AxisAlignment=Q-axis  Kp_id=0.62832  Ki_id=41.888  Kaw_id=6667  Kp_iq=1.888496  Ki_iq=41.888  Kaw_iq=2222  AxisPrio=Q-axis  ActZC=off  ActFF=on  ParamTypeFF=Constant parameters  LdFF=0.00013  LqFF=0.00038  psimFF=0.05  idVect=[-200, 0, 200]  iqVect=[-200, 0, 200]  LdMatrix=0.0002 * ones(3, 3)  LqMatrix=0.0002 * ones(3, 3)  psimMatrix=0.04 * ones(3, 3)  CPWMMode=SVM: space vector modulation  fsw=10e3
  Rate Limiter : RateLimiter  RisingSlewLimit=500  FallingSlewLimit=-800  SampleTimeMode=inherited
  Vdc : Constant  Value=800  SampleTime=Tsc
  "rpm -> rad/s [mech.]" : Gain  Gain=2*pi/60
  G : Outport  VectorParamsAs1DForOutWhenUnconnected=off
  tag scope: G=global, iMotor=global, trqDemand=global, wDemand=global
  wires:
  IPMSM Field-Oriented Control/1 -> G/1, [G]
  Vdc/1 -> IPMSM Field-Oriented Control/5
  IPMSM Field-Oriented Control/2 -> Bus Selector/1
  i_abc/1 -> IPMSM Field-Oriented Control/2
  meas/1 -> Demux1/1
  Demux1/1 -> IPMSM Field-Oriented Control/3
  Demux1/2 -> IPMSM Field-Oriented Control/4
  Bus Selector/1 -> [iMotor]  "<iabc [A]>"
  Bus Selector/2 -> [wDemand]  "<Reference>"
  Bus Selector/3 -> [trqDemand]  "<TqRef [N*m]>"
  rpm/1 -> "rpm -> rad/s [mech.]"/1
  Rate Limiter/1 -> IPMSM Field-Oriented Control/1
  "rpm -> rad/s [mech.]"/1 -> Rate Limiter/1

== system Main_Model_CB_EN_UEEE23112/Power Train/Sensing currents ==
  Current Sensor : ee_lib/Sensors & Transducers/Current Sensor (Three-Phase)
  Gain : Gain  Commented=through  Gain=1/sqrt(3)
  PS-Simulink Converter : nesl_utility/PS-Simulink Converter  PhysicalDomain=network_engine_domain  SubClassName=ps_output  LeftPortType=input  RightPortType=output  PseudoPeriodic=off  Frequencies=[]  VectorFormat=1-D array  Unit=A  AffineConversion=off
  Conn1 : PMIOPort  Side=Left
  Conn2 : PMIOPort  Port=2  Side=Right
  tag scope: i=global
  wires:
  PS-Simulink Converter/1 -> Gain/1
  Gain/1 -> [i]
  connections:
  Current Sensor/RConn1 -- PS-Simulink Converter/LConn1
  Conn2/RConn1 -- Current Sensor/RConn2
  Current Sensor/LConn1 -- Conn1/RConn1

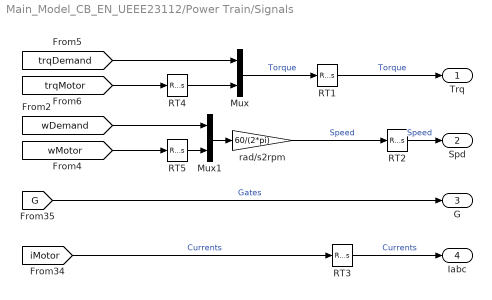
== system Main_Model_CB_EN_UEEE23112/Power Train/Signals  ==
  Mux : Mux  Inputs=2
  Mux1 : Mux  Inputs=2
  RT1 : RateTransition  OutPortSampleTime=Ts
  RT2 : RateTransition  OutPortSampleTime=Ts
  RT3 : RateTransition  OutPortSampleTime=Ts
  RT4 : RateTransition  OutPortSampleTime=Tsc
  RT5 : RateTransition  OutPortSampleTime=Tsc
  rad/s2rpm : Gain  Gain=60/(2*pi)
  Trq : Outport  VectorParamsAs1DForOutWhenUnconnected=off
  Spd : Outport  Port=2  VectorParamsAs1DForOutWhenUnconnected=off
  G : Outport  Port=3  VectorParamsAs1DForOutWhenUnconnected=off
  Iabc : Outport  Port=4  VectorParamsAs1DForOutWhenUnconnected=off
  wires:
  [trqDemand] -> Mux/1
  [G] -> G/1  "Gates"
  Mux1/1 -> rad/s2rpm/1
  Mux/1 -> RT1/1  "Torque"
  [iMotor] -> RT3/1  "Currents"
  [wDemand] -> Mux1/1
  rad/s2rpm/1 -> RT2/1  "Speed"
  [trqMotor] -> RT4/1
  [wMotor] -> RT5/1
  RT2/1 -> Spd/1  "Speed"
  RT3/1 -> Iabc/1  "Currents"
  RT4/1 -> Mux/2
  RT5/1 -> Mux1/2
  RT1/1 -> Trq/1  "Torque"
